simulink model "ILC"  (R2019a)
settings: Solver=VariableStepAuto  StartTime=0.0  StopTime=10.0  RelTol=1e-3
values from neighbouring files (symbols this model uses):
  K = (Kp + Ki*(1/s) + Kd*s) / (s + 100)    [ILC_code.m]
  Kd = 2.0    (= 2)    [ILC_code.m]
  Ki = 0.7    [ILC_code.m]
  Kp = 0.2    [ILC_code.m]
libraries: cstblocks x2, simulink x1
settings Model: Creator=capn  LastModifiedBy=emma
settings DataIOCC: ReturnWorkspaceOutputs=off
settings DebuggingCC: ArithmeticOperatorsInVariantConditions=warning
settings SFSimCC: SimUseLocalCustomCode=off
settings RTWCC: RTWUseLocalCustomCode=off
settings CodeAppCC: StateflowObjectComments=on

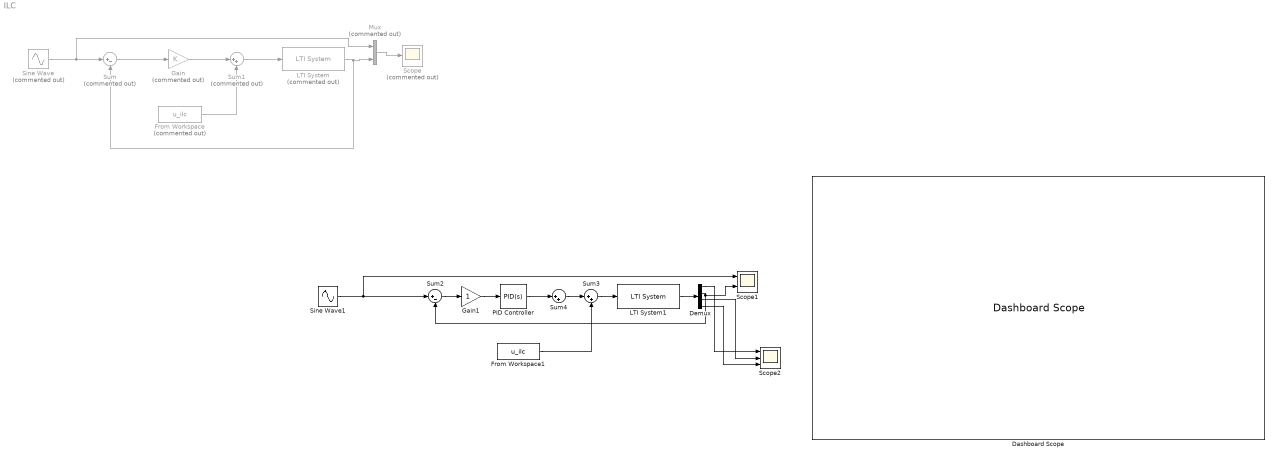
== system ILC ==
  Dashboard Scope : DashboardScope
  Demux : Demux
  From Workspace : FromWorkspace  Commented=on  VariableName=u_ilc  SampleTime=0
  From Workspace1 : FromWorkspace  VariableName=u_ilc  SampleTime=0
  Gain : Gain  Commented=on  Gain=K
  Gain1 : Gain
  LTI System : cstblocks/LTI System  Commented=on  sys=Pd  IC=[]
  LTI System1 : cstblocks/LTI System  sys=G  IC=[]
  Mux : Mux  Commented=on  Inputs=2
  PID Controller : simulink/Continuous/PID Controller  Controller=PID  Form=Parallel  TimeDomain=Continuous-time  SampleTime=-1  IntegratorMethod=Forward Euler  FilterMethod=Forward Euler  ControllerParametersSource=internal  P=Kp  I=Ki  D=Kd  UseFilter=on  N=100  TunerSelectOption=Transfer Function Based (PID Tuner App)  InitialConditionSource=internal  InitialConditionForIntegrator=0  InitialConditionForFilter=0  DifferentiatorICPrevScaledInput=0  ExternalReset=none  TrackingMode=off  Kt=1  LimitOutput=off  UpperSaturationLimit=inf  LowerSaturationLimit=-inf  LinearizeAsGain=on  AntiWindupMode=none  Kb=1  POutMin=[]  POutMax=[]  IOutMin=[]  IOutMax=[]  DOutMin=[]  DOutMax=[]  NOutMin=[]  NOutMax=[]  SumOutMin=[]  SumOutMax=[]  SaturationOutMin=[]  SaturationOutMax=[]  PParamMin=[]  PParamMax=[]  IParamMin=[]  IParamMax=[]  DParamMin=[]  DParamMax=[]  NParamMin=[]  NParamMax=[]  KbParamMin=[]  KbParamMax=[]  KtParamMin=[]  KtParamMax=[]  KbOutMin=[]  KbOutMax=[]  KtOutMin=[]  KtOutMax=[]  IntegratorOutMin=[]  IntegratorOutMax=[]  FilterOutMin=[]  FilterOutMax=[]  SumI1OutMin=[]  SumI1OutMax=[]  SumI2OutMin=[]  SumI2OutMax=[]  SumI3OutMin=[]  SumI3OutMax=[]  SumI4OutMin=[]  SumI4OutMax=[]  SumDOutMin=[]  SumDOutMax=[]  DifferentiatorOutMin=[]  DifferentiatorOutMax=[]  FilterDiffOutCoefMin=[]  FilterDiffOutCoefMax=[]  ReciprocalOutMin=[]  ReciprocalOutMax=[]  SumDenOutMin=[]  SumDenOutMax=[]  SumNumOutMin=[]  SumNumOutMax=[]  DivideOutMin=[]  DivideOutMax=[]  IntegratorContinuousStateAttributes=''  IntegratorStateMustResolveToSignalObject=off  IntegratorRTWStateStorageClass=Auto  FilterContinuousStateAttributes=''  FilterStateMustResolveToSignalObject=off  FilterRTWStateStorageClass=Auto  ParallelPVariant=InternalParameters  IdealPVariant=Disabled  IVariant=InternalParameters  DVariant=InternalParameters  IntegratorVariant=Continuous  SatVariant=Disabled  AWVariant=Passthrough  PCopyVariant=Disabled  TRVariant=Disabled  FdbkBlocksVariant=Forward  IdealPFdbkVariant=Disabled  SatFdbkVariant=Disabled  DerivativeFilterVariant=ContFilter  NVariant=InternalParameters  NCopyVariant=Disabled  FilterICVariant=InternalICsFilter  IntegratorICVariant=InternalICs  ExternalResetVariant=Disabled  TRSumVariant=Passthrough  SumFdbkVariant=Disabled  SumVariant=Sum_PID
  Scope : Scope  Commented=on
  Scope1 : Scope  NumInputPorts=2
  Scope2 : Scope  NumInputPorts=3
  Sine Wave : Sin  Commented=on  SampleTime=0
  Sine Wave1 : Sin  SampleTime=0
  Sum : Sum  Commented=on  Inputs=|+-
  Sum1 : Sum  Commented=on  Inputs=|++
  Sum2 : Sum  Inputs=|+-
  Sum3 : Sum  Inputs=|++
  Sum4 : Sum  Inputs=|++
  wires:
  Sum/1 -> Gain/1
  Gain/1 -> Sum1/1
  Sum1/1 -> LTI System/1
  Sine Wave/1 -> Mux/1, Sum/1
  From Workspace/1 -> Sum1/2
  LTI System/1 -> Mux/2, Sum/2
  Mux/1 -> Scope/1
  Sine Wave1/1 -> Sum2/1, Scope1/1
  LTI System1/1 -> Demux/1
  Demux/2 -> Scope1/2, Sum2/2
  Demux/3 -> Scope2/2
  Demux/4 -> Scope2/3
  Demux/1 -> Scope2/1
  Gain1/1 -> PID Controller/1
  Sum3/1 -> LTI System1/1
  From Workspace1/1 -> Sum3/2
  Sum2/1 -> Gain1/1
  Sum4/1 -> Sum3/1
  PID Controller/1 -> Sum4/1
